simulink model "heli_model_estim"  (R2016a)
settings: Solver=VariableStepAuto  StartTime=0.0  StopTime=10.0  RelTol=1e-3
undefined symbols (not defined in the file or in its folder): A, A_m, B, B_m, C, C_m, D, K_i, K_m, pitch, u_vec, yaw
settings Model: Creator=lukas  LastModifiedBy=lukas

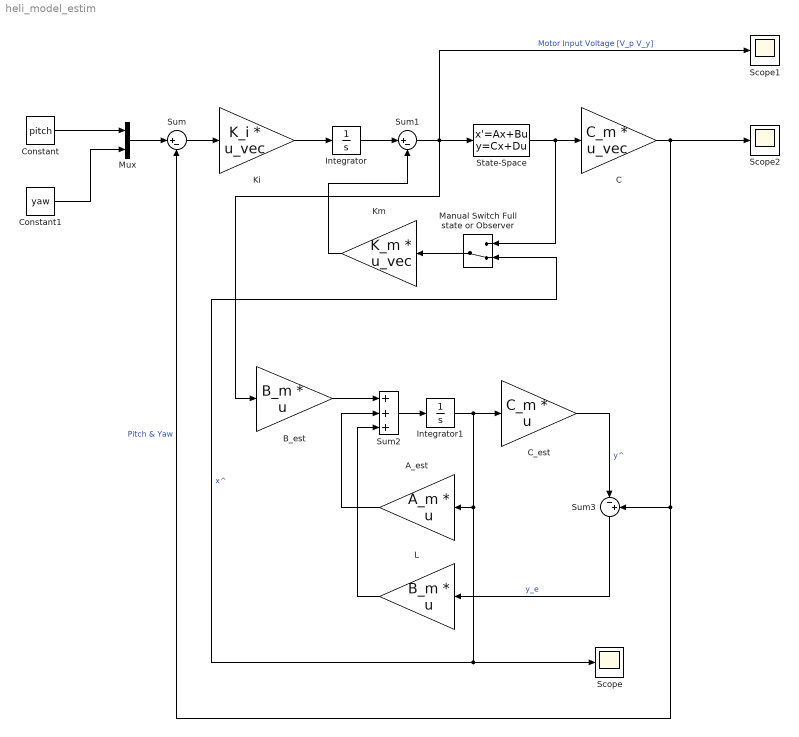
== system heli_model_estim ==
  A_est : Gain  Gain=A_m * u
  B_est : Gain  Gain=B_m * u
  C : Gain  Gain=C_m * u_vec
  C_est : Gain  Gain=C_m * u
  Constant : Constant  Value=pitch
  Constant1 : Constant  Value=yaw
  Integrator : Integrator
  Integrator1 : Integrator
  Ki : Gain  Gain=K_i * u_vec
  Km : Gain  Gain=K_m * u_vec
  L : Gain  Gain=B_m * u
  Manual Switch Full state or Observer : ManualSwitch  CurrentSetting=0
  Mux : Mux  Inputs=2
  Scope : Scope
  Scope1 : Scope
  Scope2 : Scope
  State-Space : StateSpace  A=A  B=B  C=C  D=D  X0=0
  Sum : Sum  Inputs=|+-
  Sum1 : Sum  Inputs=|+-
  Sum2 : Sum  Inputs=+++
  Sum3 : Sum  Inputs=|-+
  wires:
  Km/1 -> Sum1/2
  Manual Switch Full state or Observer/1 -> Km/1
  State-Space/1 -> Manual Switch Full state or Observer/1, C/1
  Sum1/1 -> B_est/1, Scope1/1, State-Space/1  "Motor Input Voltage [V_p V_y]"
  Integrator/1 -> Sum1/1
  Ki/1 -> Integrator/1
  Sum/1 -> Ki/1
  C/1 -> Scope2/1, Sum3/2, Sum/2  "Pitch & Yaw"
  B_est/1 -> Sum2/1
  A_est/1 -> Sum2/2
  L/1 -> Sum2/3
  Sum2/1 -> Integrator1/1
  Integrator1/1 -> C_est/1, A_est/1, Scope/1, Manual Switch Full state or Observer/2  "x^"
  C_est/1 -> Sum3/1  "y^"
  Sum3/1 -> L/1  "y_e"
  Mux/1 -> Sum/1
  Constant/1 -> Mux/1
  Constant1/1 -> Mux/2
